simulink library "Ventilation"  (Simulink 8.2)
settings: Solver=ode45  StartTime=0.0  StopTime=10.0  RelTol=1e-3
undefined symbols (not defined in the file): Ahabit, Hroom, rec, vent
settings Model: Creator=lena.frank  LastModifiedBy=drhf

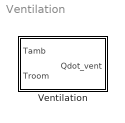
== system Ventilation ==
  Ventilation : Subsystem  mask(ventilation system with heat recovery){vent=vent, rec=rec, Vhouse=Ahabit*Hroom}
      mask prompts: vent "ventilation rate in 1/h"; rec "heat recovery (0..1)"; Vhouse "Volume of the house"
      mask help: Mechanical ventilation system with heat recovery for the simple building model (see /Load/Houses/Simpe_House).
      mask init:
      | rec = max(0,min(1,rec));
      mask Help: web(fullfile(path_carnot('help'),'Ventilation.html'),'-helpbrowser')

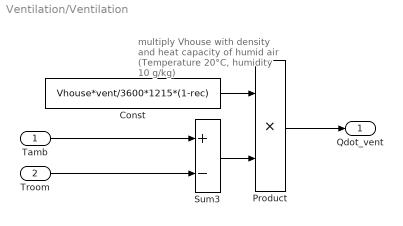
== system Ventilation/Ventilation ==
  note: multiply Vhouse with
      | density and heat capacity of humid air
      | (Temperature 20°C, humidity 10 g/kg)
  Tamb : Inport
  Troom : Inport  Port=2
  Const : Constant  Value=Vhouse*vent/3600*1215*(1-rec)
  Product : Product  RndMeth=Zero
  Sum3 : Sum  Inputs=+-  SaturateOnIntegerOverflow=on  InputSameDT=on  OutDataTypeStr=Inherit: Same as first input
  Qdot_vent : Outport
  wires:
  Troom/1 -> Sum3/2
  Sum3/1 -> Product/2
  Tamb/1 -> Sum3/1
  Product/1 -> Qdot_vent/1
  Const/1 -> Product/1
